simulink model "PII_speed"  (Simulink 7.5)
settings: Solver=ode1  SolverMode=SingleTasking  StartTime=0.0  StopTime=Inf  FixedStep=ts  RelTol=1e-3
PostLoadFcn:
  | , if any(exist('dsrtsu_mdlpostloadfcn', 'file') == [2, 3, 6]), try dsrtsu_mdlpostloadfcn('Execute', bdroot); catch fprintf('Error in PostLoadFcn (dsrtsu_mdlpostloadfcn) for model "%s":\n %s\n', bdroot, lasterr); end, end,
values from neighbouring files (symbols this model uses):
  Amp = 0    [RUN.m]
  en = 0    [RUN.m]
  f = 0.20    (= 0.2)    [RUN.m]
  g = 1    [RUN.m]
  kii = 660    [RUN.m]
  kpi = 2.0    (= 2)    [RUN.m]
  limit = 1    [RUN.m]
  nap = 0    [RUN.m]
  obc_del = 0.7    [RUN.m]
  obc_del2 = 1.3    [RUN.m]
  obc_en = 0    [RUN.m]
  obc_en1 = 0    [RUN.m]
  offset = 0    [RUN.m]
  res = 1    [RUN.m]
  res1 = 1    [RUN.m]
  start = 0    [RUN.m]
  Tf = 0.01    [RUN.m]
  Ts_i = 0.0002    [RUN.m]
  Ts_w = 0.001    [RUN.m]
undefined symbols (not defined in the file or in its folder): k1_singletons, k1k, k2_singletons, k2k, k3_singletons, k3k, kdu, Ki_singletons, Kik, ku, mf
libraries: fuzblock x15, rtilib1103 x6, simulink_extras x1
(part 1 of 2)
settings Model: DSRTSU_INTERNAL_RTI_VER=400  DSRTSU_INTERNAL_RTI_TYPE=rti1103  Creator=lab108  LastModifiedBy=zychlewicz  TunableVars=Amp,Q,Start,en,f,g,kii,kpi,n_max,n_min,nap,nb_nb,obc_del,obc_del2,obc_en,obc_en1,obc_poz,offset,p_gain,skal_u,start  TunableVarsStorageClass=Auto,Auto,Auto,Auto,Auto,Auto,Auto,Auto,Auto,Auto,Auto,Auto,Auto,Auto,Auto,Auto,Auto,Auto,Auto,Auto,Auto  TunableVarsTypeQualifier=,,,,,,,,,,,,,,,,,,,,  BufferReuse=off
settings OptimizationCC: BlockReduction=off  InlineParams=on  OptimizeBlockIOStorage=off  BufferReuse=off  ExpressionFolding=off  LocalBlockOutputs=off
settings DebuggingCC: StrictBusMsg=Warning
settings HardwareCC: ProdIntDivRoundTo=Zero  ProdEndianess=BigEndian  ProdHWDeviceType=Generic->Custom  TargetIntDivRoundTo=Zero  TargetEndianess=BigEndian  TargetHWDeviceType=Generic->Custom
settings RTWCC: SystemTargetFile=rti1103.tlc  MakeCommand=make_rti  TemplateMakefile=rti1103.tmf  Description=dSPACE DS1103 Hardware Platform  ProcessScript=rti1103_make_rtw_hook
settings STFCustomTargetCC: ParMdlRefBuildCompliant=on  GeneratePreprocessorConditionals=Disable all  SystemTargetFile=rti1103.tlc
settings GRTTargetCC: CompOptLevelCompliant=off  MatFileLogging=off  ExtModeMexFile=noextcomm
settings CustomProperty: DataType=RTWOptions_EnumType_D__dSPACE RCPHIL 73_matlab_rti1103_tlc_rti1103_1InitialSimState  Value=RUN
settings EnumStrPairs: String=RUN
settings SimEventsCC: propDiagAttribOutput=1  propDiagFcnCallOutput=1  propDiagStatOutput=0

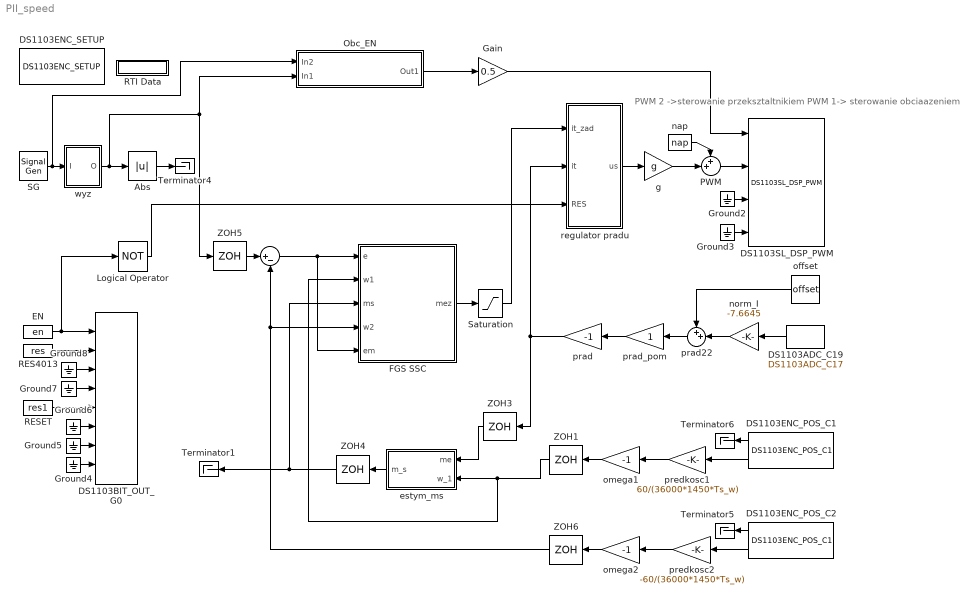
== system PII_speed ==
  note: PWM 2 ->sterowanie przeksztaltnikiem
      | PWM 1-> sterowanie obciaazeniem
  " " : Sum  Inputs=|+-  OutDataType=sfix(16)  OutScaling=2^0
  Abs : Abs  OutDataType=fixdt(1, 16)  OutScaling=2^0
  DS1103ADC_C19 : rtilib1103/DS1103 MASTER PPC/DS1103ADC_C17  SystemSampleTime=-1  ChannelNo=19  TimerAPreTrigger=0  Reserved2=[]  Reserved3=[]  Reserved4=[]  DialogFcn=gui1103adc  UnitName={ 'DS1103ADC_C' }  UnitValues={ 19 }  DSProperties=struct('RTI',struct('Version',uint32(1),'BlockType',struct('isSLSource',uint8(1),'isSLSink',uint8(0),'isHWSource',uint8(1),'isHWSink',uint8(0),'isSetup',uint8(0),'isInline',uint8(1),'isNonInline',uint8(0),'isInterrupt',uint8(0),'isChannelwise',uint8(1)),'IOBoardType','DS1103MASTER','UnitType','ADC','Identifier','ADC','DialogType','ML','BlockSet','NONE','SlaveProcessor','NONE'))
  DS1103BIT_OUT_G0 : rtilib1103/DS1103 MASTER PPC/DS1103BIT_OUT_G0  SystemSampleTime=-1  GroupNo=0  InitValue=[0 0 0 0 0 0 0 0]  TermMode=[1 1 1 1 1 1 1 1]  TermValue=[0 0 0 0 0 0 0 0]  Reserved1=[]  Reserved2=[]  Reserved3=[]  Reserved=[]  DialogFcn=gui1103bit_out  UnitName={ 'DS1103BIT_OUT_G'}  UnitValues={ 0 }  DSProperties=struct('RTI',struct('Version',uint32(1),'BlockType',struct('isSLSource',uint8(0),'isSLSink',uint8(1),'isHWSource',uint8(0),'isHWSink',uint8(1),'isSetup',uint8(0),'isInline',uint8(1),'isNonInline',uint8(0),'isInterrupt',uint8(0),'isChannelwise',uint8(0)),'IOBoardType','DS1103MASTER','UnitType','BIT','Identifier','BITOUT','DialogType','ML','BlockSet','NONE','SlaveProcessor','NONE'))
  DS1103ENC_POS_C1 : rtilib1103/DS1103 MASTER PPC/DS1103ENC_POS_C1  SystemSampleTime=-1  ChannelNo=1  PosValue=0  Reserved1=[]  Reserved2=[]  Reserved3=[]  Reserved4=[]  DialogFcn=gui1103enc_pos  UnitName={ 'DS1103ENC_POS_C' }  UnitValues={ 1 }  DSProperties=struct('RTI',struct('Version',uint32(1),'BlockType',struct('isSLSource',uint8(1),'isSLSink',uint8(0),'isHWSource',uint8(1),'isHWSink',uint8(0),'isSetup',uint8(0),'isInline',uint8(1),'isNonInline',uint8(0),'isInterrupt',uint8(0),'isChannelwise',uint8(1)),'IOBoardType','DS1103MASTER','UnitType','ENC','Identifier','ENCPOSCH','DialogType','ML','BlockSet','NONE','SlaveProcessor','NONE'))
  DS1103ENC_POS_C2 : rtilib1103/DS1103 MASTER PPC/DS1103ENC_POS_C1  SystemSampleTime=-1  ChannelNo=2  PosValue=0  Reserved1=[]  Reserved2=[]  Reserved3=[]  Reserved4=[]  DialogFcn=gui1103enc_pos  UnitName={ 'DS1103ENC_POS_C' }  UnitValues={2}  DSProperties=struct('RTI',struct('Version',uint32(1),'BlockType',struct('isSLSource',uint8(1),'isSLSink',uint8(0),'isHWSource',uint8(1),'isHWSink',uint8(0),'isSetup',uint8(0),'isInline',uint8(1),'isNonInline',uint8(0),'isInterrupt',uint8(0),'isChannelwise',uint8(1)),'IOBoardType','DS1103MASTER','UnitType','ENC','Identifier','ENCPOSCH','DialogType','ML','BlockSet','NONE','SlaveProcessor','NONE'))
  DS1103ENC_SETUP : rtilib1103/DS1103 MASTER PPC/DS1103ENC_SETUP  SystemSampleTime=-1  EncRange=2  Reserved1=[]  Reserved2=[]  Reserved3=[]  Reserved4=[]  DialogFcn=gui1103enc_setup  UnitName={ 'DS1103ENC_SETUP' }  UnitValues={ [] }  DSProperties=struct('RTI',struct('Version',uint32(1),'BlockType',struct('isSLSource',uint8(0),'isSLSink',uint8(0),'isHWSource',uint8(0),'isHWSink',uint8(0),'isSetup',uint8(0),'isInline',uint8(1),'isNonInline',uint8(0),'isInterrupt',uint8(0),'isChannelwise',uint8(0)),'IOBoardType','DS1103MASTER','UnitType','ENC','Identifier','ENCMASTER','DialogType','ML','BlockSet','NONE','SlaveProcessor','NONE'))
      settings: SignalType=[1 1 1 1 1 1 0]
  DS1103SL_DSP_PWM : rtilib1103/DS1103 SLAVE DSP/DS1103SL_DSP_PWM  SystemSampleTime=-1  Parameters=[]  TDef=[]  BoardType=[]  PwmMode=[]  Frequency=[]  InitValue=[]  TermMode=[]  TermValue=[]  Polarity=[]  DialogFcn=[]  Reserved1=[]  Reserved2=[]  Reserved3=[]  Reserved4=[]  Revision=[]  UnitName=[]  UnitValues=[]  DSProperties=struct('RTI',struct('Version',uint32(2),'BlockType',struct('isSLSource',uint8(0),'isSLSink',uint8(1),'isHWSource',uint8(0),'isHWSink',uint8(1),'isSetup',uint8(0),'isInline',uint8(1),'isNonInline',uint8(0),'isInterrupt',uint8(0),'isChannelwise',uint8(0)),'IOBoardType','DS1103SLAVE','UnitType','PWM','Identifier','PWM','DialogType','ML','BlockSet','NONE','SlaveProcessor','F240'))  RTIBlockInterface=struct('InputPortsActive',[1 1 1 1],'InputPortsWidth',int32([2 1 2 2]),'InputPortsName',{{['PWM Channel 1'],['PWM Channel 2'],['PWM Channel 3'],['PWM Channel 4']}},'IWork',{{{'',uint32(4)}}},'DialogFcn','rti1103slavepwmgui','InitLevel',1,'BlockDisplay',{{'','auto'}},'IconTransparency','on','MultiSFcn',4,'BlockName',struct('Token',{{'DS1103SL_DSP_PWM'}}))  RTIBlockParameters=struct('PWMSymmetryMode',{{1,'OFF',[]}},'PWMFrequency',{{'12000','OFF',[]}},'PWMPolarityMode',{{[1 1 1 1 1],'OFF',[]}},'ChannelNo',{{[1 2 3 4],'OFF',[]}},'SuspendModeInit',{{[1 0 1 1 1],'OFF',[]}},'TTLModeInit',{{[2 2 2 2 2],'OFF',[]}},'DutyCycleInitValueCh1',{{'0.5','OFF',[]}},'DutyCycleInitValueCh2',{{'0.5','OFF',[]}},'DutyCycleInitValueCh3',{{'0.5','OFF',[]}},'DutyCycleInitValueCh4',{{'0.5','OFF',[]}},'DutyCycleInitValueCh5',{{'0.5','OFF',[]}},'EnablePWMStop',{{[1 1 1 1 0],'OFF',[]}},'SuspendModeTerm',{{[1 0 1 1 1],'OFF',[]}},'TTLModeTerm',{{[2 2 2 2 2],'OFF',[]}},'DutyCycleTermValueCh1',{{'0.5','OFF',[]}},'DutyCycleTermValueCh2',{{'0.5','OFF',[]}},'DutyCycleTermValueCh3',{{'0.5','OFF',[]}},'DutyCycleTermValueCh4',{{'0.5','OFF',[]}},'DutyCycleTermValueCh5',{{'0.5','OFF',[]}},'TLCFileName',{{'rti1103pwm','OFF',[]}})  RTISFcnParameters=struct('PWMSymmetryMode','double','PWMFrequency','double','PWMPolarityMode','double','ChannelNo','double','SuspendModeInit','double','TTLModeInit','double','DutyCycleInitValueCh1','double','DutyCycleInitValueCh2','double','DutyCycleInitValueCh3','double','DutyCycleInitValueCh4','double','EnablePWMStop','double','SuspendModeTerm','double','TTLModeTerm','double','DutyCycleTermValueCh1','double','DutyCycleTermValueCh2','double','DutyCycleTermValueCh3','double','DutyCycleTermValueCh4','double','TLCFileName','char')  RTIBlockParaDefault=struct('PWMSymmetryMode',1,'PWMFrequency',100,'PWMPolarityMode',[1 1 1 1 1],'ChannelNo',[1 2 3 4],'SuspendModeInit',[1 1 1 1 1],'TTLModeInit',[2 2 2 2 2],'DutyCycleInitValueCh1',0.5,'DutyCycleInitValueCh2',0.5,'DutyCycleInitValueCh3',0.5,'DutyCycleInitValueCh4',0.5,'DutyCycleInitValueCh5',0.5,'EnablePWMStop',[1 1 1 1 0],'SuspendModeTerm',[1 1 1 1 1],'TTLModeTerm',[2 2 2 2 2],'DutyCycleTermValueCh1',0.5,'DutyCycleTermValueCh2',0.5,'DutyCycleTermValueCh3',0.5,'DutyCycleTermValueCh4',0.5,'DutyCycleTermValueCh5',0.5,'TLCFileName','rti1103pwm')
  EN : Constant  Value=en  OutDataTypeMode=boolean  OutDataType=fixdt(1, 16)  OutScaling=2^0  OutDataTypeStr=boolean
  FGS SSC : Subsystem
      mask Display:
      | port_label('input', 1, 'error', 'texmode', 'on')
      | port_label('input', 2, '\omega_1', 'texmode', 'on')
      | port_label('input', 3, 'm_s', 'texmode', 'on')
      | port_label('input', 4, '\omega_2', 'texmode', 'on')
      | port_label('input', 5, '\omega_{refm} - \omega_1', 'texmode', 'on')
      | port_label('output', 1, 'm_{ez}', 'texmode', 'on')
      | color('red')
      | disp('FGS SSC')
      | color('blue')
      | plot(gaussmf([-1:0.0001:1],[1 0]))
  Gain : Gain  Gain=0.5  ParameterDataType=sfix(16)  ParameterScaling=2^0  OutDataType=sfix(16)  OutScaling=2^0
  Ground{2..8} (7 alike) : Ground
  Logical Operator : Logic  Operator=NOT  AllPortsSameDT=off  OutDataTypeMode=boolean  LogicDataType=fixdt(0, 8)  OutDataTypeStr=boolean
  Obc_EN : Subsystem
  PWM : Sum  Inputs=++|  OutDataType=sfix(16)  OutScaling=2^0
  RES4013 : Constant  Value=res  OutDataTypeMode=boolean  OutDataType=fixdt(1, 16)  OutScaling=2^0  OutDataTypeStr=boolean
  RESET : Constant  Value=res1  OutDataTypeMode=boolean  OutDataType=fixdt(1, 16)  OutScaling=2^0  OutDataTypeStr=boolean
  RTI Data : Subsystem  Tag=struct('RTIDataServer',struct('RTIDataServerVs','2','RTIModelDescription','struct(''main'',''PII_speed'',''sub'','''',''isMp'',0)'))  LoadFcn="if exist('rtidc'), try,  rtidc('DataHostBlockClbLoad', gcbh); catch, disp(['Warning: ''LoadFcn'' for RTI Data block failed: ' lasterr]); end, end,"
      settings: CopyFcn="if exist('rtidc'), try,  rtidc('DataHostBlockClbCopy', gcbh); catch, disp(['Warning: ''CopyFcn'' for RTI Data block failed: ' lasterr]); end, end,"  DeleteFcn="if exist('rtidc'), try,  rtidc('DataHostBlockClbDelete', gcbh); catch, disp(['Warning: ''DeleteFcn'' for RTI Data block failed: ' lasterr]); end, end,"  ModelCloseFcn="if exist('rtidc'), try,  rtidc('DataHostBlockClbModelClose', gcbh); catch, disp(['Warning: ''ModelCloseFcn'' for RTI Data block failed: ' lasterr]); end, end,"  PreSaveFcn="if exist('rtidc'), try,  rtidc('DataHostBlockClbPreSave', gcbh); catch, disp(['Warning: ''PreSaveFcn'' for RTI Data block failed: ' lasterr]); end, end,"  PostSaveFcn="if exist('rtidc'), try,  rtidc('DataHostBlockClbPostSave', gcbh); catch, disp(['Warning: ''PostSaveFcn'' for RTI Data block failed: ' lasterr]); end, end,"  NameChangeFcn="if exist('rtidc'), try,  rtidc('DataHostBlockClbNameChange', gcbh); catch, disp(['Warning: ''NameChangeFcn'' for RTI Data block failed: ' lasterr]); end, end,"
      mask Type: RTI_DATA_HOST
      mask Description:
      | RTI Data Block.
      | This block is used by RTI to store internal model-dependent data.
      | Please keep this block on the root level of the model. Deleting this block will result in data loss.
      | 
      | NEVER DELETE OR COPY THIS BLOCK!
      mask Help:
      | RTI Data Block.
      | This block is used by RTI to store internal model-dependent data.
      | Please keep this block on the root level of the model. Deleting this block will result in data loss.
      | 
      | NEVER DELETE OR COPY THIS BLOCK!
      mask Display:
      | text(0.5, 0.5, 'RTI Data', 'HorizontalAlignment', 'center');
      | plot([1 0]);
  SG : SignalGenerator  WaveForm=square  Amplitude=Amp  Frequency=f
  Saturation : Saturate  UpperLimit=limit  LowerLimit=-limit
  Terminator{1,4..6} (4 alike) : Terminator
  ZOH{1,3..6} (5 alike) : ZeroOrderHold  SampleTime=Ts_w
  estym_ms : Subsystem
  g : Gain  Gain=g  ParameterDataType=fixdt(1, 16)  ParameterScaling=2^0  OutDataType=fixdt(1, 16)  OutScaling=2^0
  nap : Constant  Value=nap  OutDataType=sfix(16)  OutScaling=2^0
  norm_I : Gain  Gain=-7.6645  ParameterDataType=fixdt(1, 16)  ParameterScaling=2^0  OutDataType=fixdt(1, 16)  OutScaling=2^0
  offset : Constant  Value=offset  OutDataType=sfix(16)  OutScaling=2^0
  omega1 : Gain  Gain=-1  OutDataTypeMode=double  OutDataTypeStr=double  SampleTime=Ts_w  SaturateOnIntegerOverflow=on  ParamDataTypeStr=Inherit: Same as input
  omega2 : Gain  Gain=-1  OutDataTypeMode=double  OutDataTypeStr=double  SampleTime=Ts_w  SaturateOnIntegerOverflow=on  ParamDataTypeStr=Inherit: Same as input
  prad : Gain  Gain=-1  OutDataTypeMode=double  OutDataTypeStr=double  SampleTime=Ts_i  SaturateOnIntegerOverflow=on  ParamDataTypeStr=Inherit: Same as input
  prad22 : Sum  Inputs=++|  OutDataType=sfix(16)  OutScaling=2^0
  prad_pom : Gain  OutDataTypeMode=double  OutDataTypeStr=double  SampleTime=Ts_i  SaturateOnIntegerOverflow=on  ParamDataTypeStr=Inherit: Same as input
  predkosc1 : Gain  Gain=60/(36000*1450*Ts_w)  OutDataTypeMode=double  OutDataTypeStr=double  SampleTime=Ts_w  SaturateOnIntegerOverflow=on  ParamDataTypeStr=Inherit: Same as input
  predkosc2 : Gain  Gain=-60/(36000*1450*Ts_w)  OutDataTypeMode=double  OutDataTypeStr=double  SampleTime=Ts_w  SaturateOnIntegerOverflow=on  ParamDataTypeStr=Inherit: Same as input
  regulator pradu : Subsystem
  wyz : Subsystem
  wires:
  EN/1 -> DS1103BIT_OUT_G0/1, Logical Operator/1
  RESET/1 -> DS1103BIT_OUT_G0/5
  RES4013/1 -> DS1103BIT_OUT_G0/2
  DS1103ADC_C19/1 -> norm_I/1
  offset/1 -> prad22/1
  norm_I/1 -> prad22/2
  DS1103ENC_POS_C1/2 -> predkosc1/1
  prad22/1 -> prad_pom/1
  DS1103ENC_POS_C2/2 -> predkosc2/1
  nap/1 -> PWM/1
  regulator pradu/1(us) -> g/1
  PWM/1 -> DS1103SL_DSP_PWM/2
  g/1 -> PWM/2
  SG/1 -> wyz/1(I), Obc_EN/1(In2)
  predkosc2/1 -> omega2/1
  predkosc1/1 -> omega1/1
  wyz/1(O) -> Abs/1, Obc_EN/2(In1), ZOH5/1
  Ground2/1 -> DS1103SL_DSP_PWM/3
  Ground3/1 -> DS1103SL_DSP_PWM/4
  Ground4/1 -> DS1103BIT_OUT_G0/8
  Ground5/1 -> DS1103BIT_OUT_G0/7
  Ground6/1 -> DS1103BIT_OUT_G0/6
  Ground7/1 -> DS1103BIT_OUT_G0/4
  Ground8/1 -> DS1103BIT_OUT_G0/3
  Abs/1 -> Terminator4/1
  DS1103ENC_POS_C2/1 -> Terminator5/1
  DS1103ENC_POS_C1/1 -> Terminator6/1
  Logical Operator/1 -> regulator pradu/3(RES)
  prad/1 -> regulator pradu/2(it), ZOH3/1
  Obc_EN/1(Out1) -> Gain/1
  Gain/1 -> DS1103SL_DSP_PWM/1
  ZOH3/1 -> estym_ms/1(me)
  omega1/1 -> ZOH1/1
  ZOH1/1 -> estym_ms/2(w_1), FGS SSC/2(w1)
  prad_pom/1 -> prad/1
  omega2/1 -> ZOH6/1
  estym_ms/1(m_s) -> ZOH4/1
  Saturation/1 -> regulator pradu/1(it_zad)
  FGS SSC/1(mez) -> Saturation/1
  ZOH4/1 -> Terminator1/1, FGS SSC/3(ms)
  ZOH6/1 -> FGS SSC/4(w2), " "/2
  ZOH5/1 -> " "/1
  " "/1 -> FGS SSC/1(e), FGS SSC/5(em)

== system PII_speed/FGS SSC ==
  e : Inport
  w1 : Inport  Port=2
  ms : Inport  Port=3
  w2 : Inport  Port=4
  em : Inport  Port=5
  FGS : Subsystem
      mask Display:
      | port_label('output',1,'K_i^{fuzzy}','texmode','on')
      | port_label('output',2,'k_1^{fuzzy}','texmode','on')
      | port_label('output',3,'k_2^{fuzzy}','texmode','on')
      | port_label('output',4,'k_3^{fuzzy}','texmode','on')
      | port_label('input',1,'error','texmode','on')
  Integrator : Integrator
  Product{1..2,5..6} (4 alike) : Product
  Sum1 : Sum  Inputs=++|
  Sum7 : Sum  Inputs=|+-
  Sum9 : Sum  Inputs=++|
  mez : Outport
  wires:
  Sum9/1 -> Sum7/2
  Sum1/1 -> Sum9/2
  Product6/1 -> Sum1/2
  Product2/1 -> Sum9/1
  w2/1 -> Product6/1
  ms/1 -> Product5/1
  w1/1 -> Product2/1
  Sum7/1 -> mez/1
  Product1/1 -> Sum7/1
  Integrator/1 -> Product1/1
  e/1 -> Integrator/1
  Product5/1 -> Sum1/1
  em/1 -> FGS/1(e)
  FGS/1(Kifuzzy) -> Product1/2
  FGS/2(k1fuzzy) -> Product2/2
  FGS/4(k3fuzzy) -> Product6/2
  FGS/3(k2fuzzy) -> Product5/2

== system PII_speed/Obc_EN ==
  In2 : Inport
  In1 : Inport  Port=2
  Abs : Abs  OutDataType=fixdt(1, 16)  OutScaling=2^0
  Add : Sum  Inputs=+-  OutDataType=fixdt(1, 16)  OutScaling=2^-10
  Bus Creator : BusCreator  Inputs=2
  Gain : Gain  Gain=-1  ParameterDataType=sfix(16)  ParameterScaling=2^0  OutDataType=sfix(16)  OutScaling=2^0
  Obc_en : Step  Time=0  After=obc_en  SampleTime=0
  Obc_en1 : Step  Time=0  After=obc_en1  SampleTime=0
  Obc_poziom : Lookup  InputValues=[0,0.25,0.3,0.4,0.5,0.6,0.75,1]  Table=[-1,-1,-0.78,-0.4,-0.3,-0.24,-0.18,-0.13]  OutDataType=fixdt(1, 16)  OutScaling=2^0
  Product : Product  Inputs=3  OutDataType=sfix(16)  OutScaling=2^0  RndMeth=Zero
  Sign : Signum
  Sign1 : Signum
  TD : TransportDelay  DelayTime=obc_del  BufferSize=60000
  TD1 : TransportDelay  DelayTime=obc_del2  BufferSize=60000
  Out1 : Outport
  wires:
  Obc_en/1 -> Product/1
  Product/1 -> Bus Creator/1
  In1/1 -> Gain/1
  Bus Creator/1 -> Out1/1
  TD/1 -> Sign/1, TD1/1
  Sign/1 -> Add/1
  Gain/1 -> TD/1
  TD1/1 -> Sign1/1
  Sign1/1 -> Add/2
  Add/1 -> Product/2
  Abs/1 -> Obc_poziom/1
  Obc_poziom/1 -> Product/3
  In2/1 -> Abs/1
  Obc_en1/1 -> Bus Creator/2

== system PII_speed/RTI Data ==
  RTI Data Store : Subsystem  Tag="struct('private',struct('version',struct('dsVer',uint32(2),'dsVerCreation',uint32(2),'RTI',struct('ver','6.4','type','RTI1103')),'access',struct('type','Model','isPerm',1,'created',['17-Sep-2010 12:08:45'],'modified',['21-Jan-2016 14:22:11'],'location','')),'public',struct('main',struct('data',[]),'sub',struct('name',{{'PII_speed'}},'data',{{struct('TH',struct('thTaskInfo',struct('taskType',{'TIMER','HWINT','TMRINT','SWINT','GLINT'},'tasksNumOf',{1,0,0,0,0},'srcIds',{{'TIMERA'},{},{},{},{}},'taskNames',{{['Timer Task 1']},{},{},{},{}})),'th_tc',struct('dataType','TASK','taskGroupId','','taskGroupList',{{}},'taskSchedulingPolicy','FCFS','taskType','TIMER','blkh',-1,'srcId','TIMERA','srcSgnName',['Timer A interrupt'],'srcCpuName','','taskName',['Timer Task 1  [0.0001] s'],'taskNameDisplayExt','','smplTime',0.0001,'smplTimeOffs',0,'hasFixedPriority',0,'priority',1,'hasFixedOvc',0,'ovcType',1,'ovcMax',1),'tc_th',struct('dataType','TASK','taskGroupId','','taskGroupList',{{}},'taskSchedulingPolicy','FCFS','taskType','TIMER','blkh',-1,'srcId','TIMERA','srcSgnName',['Timer A interrupt'],'srcCpuName','','taskName',['Timer Task 1  [0.0001] s'],'taskNameDisplayExt','','smplTime',0.0001,'smplTimeOffs',0,'hasFixedPriority',0,'priority',1,'hasFixedOvc',0,'ovcType',1,'ovcMax',1))}})))"
      mask Type: RTI_DATA_STORE
      mask Description:
      | RTI Data Store Block. This block is used by RTI to store internal model dependent data. Deleting this block will result in data loss.
      | 
      | NEVER DELETE, COPY, OR MODIFY THIS BLOCK!
      mask Help:
      | RTI Data Store Block. This block is used by RTI to store internal model dependent data. Deleting this block will result in data loss.
      | 
      | NEVER DELETE, COPY, OR MODIFY THIS BLOCK!
      mask Display: text(0.5, 0.5, ' ', 'HorizontalAlignment', 'center');

== system PII_speed/estym_ms ==
  me : Inport
  w_1 : Inport  Port=2
  Transfer Fcn1 : TransferFcn  Numerator=[0.203 0]  Denominator=[Tf 1]
  Transfer Fcn2 : TransferFcn  Denominator=[Tf 1]
  ms_est : Sum  Inputs=-+  OutDataType=sfix(16)  OutScaling=2^0
  m_s : Outport
  wires:
  ms_est/1 -> m_s/1
  me/1 -> Transfer Fcn2/1
  w_1/1 -> Transfer Fcn1/1
  Transfer Fcn2/1 -> ms_est/2
  Transfer Fcn1/1 -> ms_est/1

== system PII_speed/regulator pradu ==
  it_zad : Inport  SampleTime=Ts_i
  it : Inport  Port=2  SampleTime=Ts_i
  RES : Inport  Port=3  SampleTime=Ts_i
  Continous-time integrator : Integrator  ExternalReset=level  LimitOutput=on  UpperSaturationLimit=0.52  LowerSaturationLimit=-0.52
  KI : Gain  Gain=kii  SampleTime=Ts_i  SaturateOnIntegerOverflow=on  OutDataTypeStr=Inherit: Same as input  ParamDataTypeStr=Inherit: Same as input
  Kp : Gain  Gain=kpi  SampleTime=Ts_i  SaturateOnIntegerOverflow=on  OutDataTypeStr=Inherit: Same as input  ParamDataTypeStr=Inherit: Same as input
  Saturation : Saturate  UpperLimit=0.52  LowerLimit=-0.52  OutDataType=fixdt(1, 16)  OutScaling=2^0
  Sum1 : Sum  Inputs=|+-  SampleTime=Ts_i  SaturateOnIntegerOverflow=on  InputSameDT=on  OutDataTypeStr=Inherit: Same as first input
  Sum2 : Sum  SampleTime=Ts_i  SaturateOnIntegerOverflow=on  InputSameDT=on  OutDataTypeStr=Inherit: Same as first input
  offset : Constant  Value=0.5  OutDataType=sfix(16)  OutScaling=2^0  SampleTime=Ts_i
  prad : Sum  Inputs=++|  OutDataType=sfix(16)  OutScaling=2^0  SampleTime=Ts_i
  us : Outport
  wires:
  Kp/1 -> Sum2/1
  Sum2/1 -> Saturation/1
  Sum1/1 -> Kp/1, KI/1
  it/1 -> Sum1/2
  it_zad/1 -> Sum1/1
  RES/1 -> Continous-time integrator/2
  offset/1 -> prad/1
  prad/1 -> us/1
  KI/1 -> Continous-time integrator/1
  Continous-time integrator/1 -> Sum2/2
  Saturation/1 -> prad/2

== system PII_speed/wyz ==
  I : Inport
  HC : HitCross  HitCrossingDirection=rising
  LO : Logic  AllPortsSameDT=off  OutDataTypeMode=boolean  LogicDataType=fixdt(0, 8)  OutDataTypeStr=boolean
  LO3 : Logic  Operator=NOT  AllPortsSameDT=off
  S : Constant  Value=0  OutDataTypeMode=boolean  OutDataTypeStr=boolean
  S-R Flip-Flop : simulink_extras/Flip Flops/S-R Flip-Flop  SystemSampleTime=-1  initial_condition=0
  Start : Constant  Value=start
  Switch : Switch  Criteria=u2 ~= 0  OutDataType=fixdt(1, 16)  OutScaling=2^0
  Terminator5 : Terminator
  O : Outport
  wires:
  Start/1 -> LO3/1, LO/2
  HC/1 -> LO/1
  LO/1 -> S-R Flip-Flop/1
  LO3/1 -> S-R Flip-Flop/2
  Switch/1 -> O/1
  S/1 -> Switch/3
  S-R Flip-Flop/1 -> Switch/2
  I/1 -> HC/1, Switch/1
  S-R Flip-Flop/2 -> Terminator5/1

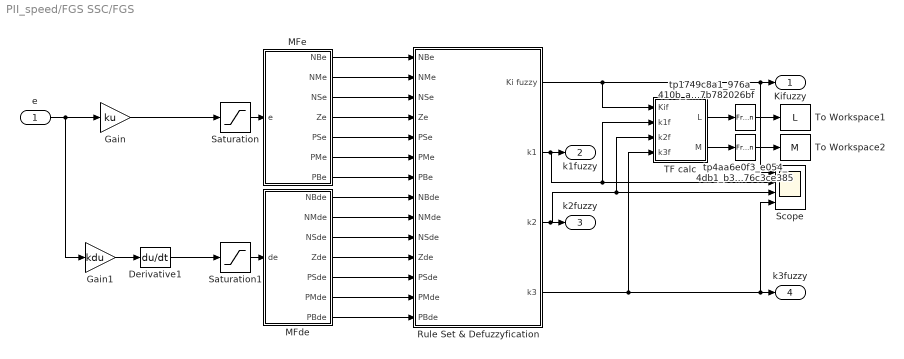
== system PII_speed/FGS SSC/FGS ==
  e : Inport
  Derivative1 : Derivative
  Gain : Gain  Gain=ku
  Gain1 : Gain  Gain=kdu
  MFde : Subsystem
  MFe : Subsystem
  Rule Set & Defuzzyfication : Subsystem
  Saturation : Saturate  UpperLimit=1  LowerLimit=-1
  Saturation1 : Saturate  UpperLimit=1  LowerLimit=-1
  Scope : Scope  NumInputPorts=4
      settings: TimeRange=20  YMin=27.01~10.375~2.85~0.061  YMax=27.08~10.42~3.2~0.0655  SaveName=data2  DataFormat=Array
  TF calc : Subsystem
  To Workspace1 : ToWorkspace  VariableName=L  SampleTime=-1  SaveFormat=Array
  To Workspace2 : ToWorkspace  VariableName=M  SampleTime=-1  SaveFormat=Array
  tp1749c8a1_976a_410b_a3f7_9c7b782026bf : FrameConversion  OutFrame=Sample-based
  tp4aa6e0f3_e054_4db1_b332_b1b76c3ce385 : FrameConversion
  Kifuzzy : Outport
  k1fuzzy : Outport  Port=2
  k2fuzzy : Outport  Port=3
  k3fuzzy : Outport  Port=4
  wires:
  Rule Set & Defuzzyfication/1(Ki fuzzy) -> TF calc/1(Kif), Kifuzzy/1, Scope/1
  MFde/7(PBde) -> Rule Set & Defuzzyfication/14(PBde)
  MFde/6(PMde) -> Rule Set & Defuzzyfication/13(PMde)
  MFde/5(PSde) -> Rule Set & Defuzzyfication/12(PSde)
  MFde/4(Zde) -> Rule Set & Defuzzyfication/11(Zde)
  MFde/3(NSde) -> Rule Set & Defuzzyfication/10(NSde)
  MFde/2(NMde) -> Rule Set & Defuzzyfication/9(NMde)
  MFde/1(NBde) -> Rule Set & Defuzzyfication/8(NBde)
  MFe/7(PBe) -> Rule Set & Defuzzyfication/7(PBe)
  MFe/6(PMe) -> Rule Set & Defuzzyfication/6(PMe)
  MFe/5(PSe) -> Rule Set & Defuzzyfication/5(PSe)
  MFe/4(Ze) -> Rule Set & Defuzzyfication/4(Ze)
  MFe/3(NSe) -> Rule Set & Defuzzyfication/3(NSe)
  MFe/2(NMe) -> Rule Set & Defuzzyfication/2(NMe)
  MFe/1(NBe) -> Rule Set & Defuzzyfication/1(NBe)
  Gain/1 -> Saturation/1
  e/1 -> Gain/1, Gain1/1
  Rule Set & Defuzzyfication/3(k2) -> Scope/3, TF calc/3(k2f), k2fuzzy/1
  Rule Set & Defuzzyfication/4(k3) -> Scope/4, k3fuzzy/1, TF calc/4(k3f)
  Rule Set & Defuzzyfication/2(k1) -> Scope/2, TF calc/2(k1f), k1fuzzy/1
  Saturation/1 -> MFe/1(e)
  Saturation1/1 -> MFde/1(de)
  Gain1/1 -> Derivative1/1
  Derivative1/1 -> Saturation1/1
  TF calc/1(L) -> tp1749c8a1_976a_410b_a3f7_9c7b782026bf/1
  tp1749c8a1_976a_410b_a3f7_9c7b782026bf/1 -> To Workspace1/1
  TF calc/2(M) -> tp4aa6e0f3_e054_4db1_b332_b1b76c3ce385/1
  tp4aa6e0f3_e054_4db1_b332_b1b76c3ce385/1 -> To Workspace2/1

== system PII_speed/RTI Data/RTI Data Store ==
  RTI Data Store : Subsystem
      mask Type: RTI_DATA_STORE
      mask Description:
      | RTI Data Store Block. This block is used by RTI to store internal model dependent data. Deleting this block will result in data loss.
      | 
      | NEVER DELETE, COPY, OR MODIFY THIS BLOCK!
      mask Help:
      | RTI Data Store Block. This block is used by RTI to store internal model dependent data. Deleting this block will result in data loss.
      | 
      | NEVER DELETE, COPY, OR MODIFY THIS BLOCK!
      mask Display: text(0.5, 0.5, ' ', 'HorizontalAlignment', 'center');

== system PII_speed/FGS SSC/FGS/MFde ==
  de : Inport
  Gaussian MF : fuzblock/Membership  Functions/Gaussian MF  sigma=sigma  mu=mf(1)
  Gaussian MF1 : fuzblock/Membership  Functions/Gaussian MF  sigma=sigma  mu=mf(2)
  Gaussian MF2 : fuzblock/Membership  Functions/Gaussian MF  sigma=sigma  mu=mf(3)
  Gaussian MF3 : fuzblock/Membership  Functions/Gaussian MF  sigma=sigma  mu=mf(4)
  Gaussian MF4 : fuzblock/Membership  Functions/Gaussian MF  sigma=sigma  mu=mf(5)
  Gaussian MF5 : fuzblock/Membership  Functions/Gaussian MF  sigma=sigma  mu=mf(6)
  Gaussian MF6 : fuzblock/Membership  Functions/Gaussian MF  sigma=sigma  mu=mf(7)
  NBde : Outport
  NMde : Outport  Port=2
  NSde : Outport  Port=3
  Zde : Outport  Port=4
  PSde : Outport  Port=5
  PMde : Outport  Port=6
  PBde : Outport  Port=7
  wires:
  Gaussian MF3/1 -> Zde/1
  de/1 -> Gaussian MF3/1, Gaussian MF2/1, Gaussian MF/1, Gaussian MF1/1, Gaussian MF4/1, Gaussian MF6/1, Gaussian MF5/1
  Gaussian MF2/1 -> NSde/1
  Gaussian MF5/1 -> PMde/1
  Gaussian MF4/1 -> PSde/1
  Gaussian MF6/1 -> PBde/1
  Gaussian MF1/1 -> NMde/1
  Gaussian MF/1 -> NBde/1

== system PII_speed/FGS SSC/FGS/MFe ==
  e : Inport
  Gaussian MF : fuzblock/Membership  Functions/Gaussian MF  SystemSampleTime=-1  sigma=sigma  mu=mf(1)
  Gaussian MF1 : fuzblock/Membership  Functions/Gaussian MF  SystemSampleTime=-1  sigma=sigma  mu=mf(2)
  Gaussian MF2 : fuzblock/Membership  Functions/Gaussian MF  SystemSampleTime=-1  sigma=sigma  mu=mf(3)
  Gaussian MF3 : fuzblock/Membership  Functions/Gaussian MF  SystemSampleTime=-1  sigma=sigma  mu=mf(4)
  Gaussian MF4 : fuzblock/Membership  Functions/Gaussian MF  SystemSampleTime=-1  sigma=sigma  mu=mf(5)
  Gaussian MF5 : fuzblock/Membership  Functions/Gaussian MF  SystemSampleTime=-1  sigma=sigma  mu=mf(6)
  Gaussian MF6 : fuzblock/Membership  Functions/Gaussian MF  SystemSampleTime=-1  sigma=sigma  mu=mf(7)
  Gaussian MF7 : fuzblock/Membership  Functions/Gaussian MF  SystemSampleTime=-1  sigma=1  mu=1
  NBe : Outport
  NMe : Outport  Port=2
  NSe : Outport  Port=3
  Ze : Outport  Port=4
  PSe : Outport  Port=5
  PMe : Outport  Port=6
  PBe : Outport  Port=7
  wires:
  Gaussian MF3/1 -> Ze/1
  e/1 -> Gaussian MF3/1, Gaussian MF2/1, Gaussian MF1/1, Gaussian MF/1, Gaussian MF4/1, Gaussian MF6/1, Gaussian MF5/1
  Gaussian MF2/1 -> NSe/1
  Gaussian MF5/1 -> PMe/1
  Gaussian MF4/1 -> PSe/1
  Gaussian MF6/1 -> PBe/1
  Gaussian MF1/1 -> NMe/1
  Gaussian MF/1 -> NBe/1

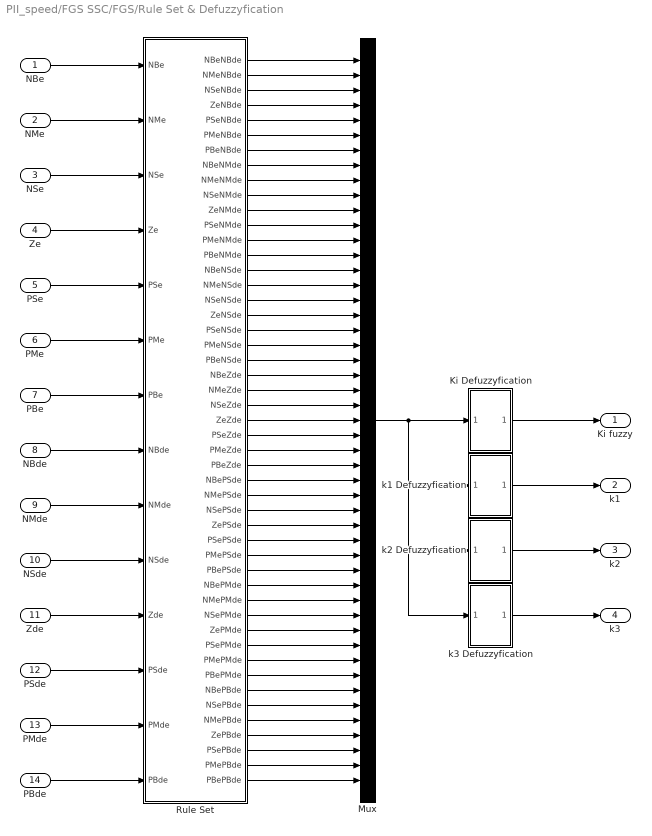
== system PII_speed/FGS SSC/FGS/Rule Set & Defuzzyfication ==
  NBe : Inport
  NMe : Inport  Port=2
  NSe : Inport  Port=3
  Ze : Inport  Port=4
  PSe : Inport  Port=5
  PMe : Inport  Port=6
  PBe : Inport  Port=7
  NBde : Inport  Port=8
  NMde : Inport  Port=9
  NSde : Inport  Port=10
  Zde : Inport  Port=11
  PSde : Inport  Port=12
  PMde : Inport  Port=13
  PBde : Inport  Port=14
  Ki Defuzzyfication : Subsystem
  Mux : Mux  Inputs=49
  Rule Set : Subsystem
  k1 Defuzzyfication : Subsystem
  k2 Defuzzyfication : Subsystem
  k3 Defuzzyfication : Subsystem
  Ki fuzzy : Outport
  k1 : Outport  Port=2
  k2 : Outport  Port=3
  k3 : Outport  Port=4
  wires:
  Mux/1 -> k1 Defuzzyfication/1(In1), k3 Defuzzyfication/1(In1), k2 Defuzzyfication/1(In1), Ki Defuzzyfication/1(In1)
  Rule Set/32(ZePSde) -> Mux/32
  Rule Set/43(NBePBde) -> Mux/43
  Rule Set/31(NSePSde) -> Mux/31
  Rule Set/33(PSePSde) -> Mux/33
  Rule Set/24(NSeZde) -> Mux/24
  Rule Set/46(ZePBde) -> Mux/46
  Rule Set/28(PBeZde) -> Mux/28
  Rule Set/49(PBePBde) -> Mux/49
  Rule Set/48(PMePBde) -> Mux/48
  Rule Set/39(ZePMde) -> Mux/39
  Rule Set/44(NSePBde) -> Mux/44
  Rule Set/35(PBePSde) -> Mux/35
  Rule Set/29(NBePSde) -> Mux/29
  Rule Set/40(PSePMde) -> Mux/40
  Rule Set/45(NMePBde) -> Mux/45
  Rule Set/27(PMeZde) -> Mux/27
  Rule Set/23(NMeZde) -> Mux/23
  Rule Set/25(ZeZde) -> Mux/25
  Rule Set/26(PSeZde) -> Mux/26
  Rule Set/34(PMePSde) -> Mux/34
  Rule Set/47(PSePBde) -> Mux/47
  Rule Set/37(NMePMde) -> Mux/37
  Rule Set/42(PBePMde) -> Mux/42
  Rule Set/41(PMePMde) -> Mux/41
  Rule Set/36(NBePMde) -> Mux/36
  Rule Set/30(NMePSde) -> Mux/30
  Rule Set/38(NSePMde) -> Mux/38
  Rule Set/22(NBeZde) -> Mux/22
  Rule Set/21(PBeNSde) -> Mux/21
  Rule Set/20(PMeNSde) -> Mux/20
  Rule Set/15(NBeNSde) -> Mux/15
  Rule Set/12(PSeNMde) -> Mux/12
  Rule Set/8(NBeNMde) -> Mux/8
  Rule Set/7(PBeNBde) -> Mux/7
  Rule Set/3(NSeNBde) -> Mux/3
  Rule Set/1(NBeNBde) -> Mux/1
  Rule Set/19(PSeNSde) -> Mux/19
  Rule Set/4(ZeNBde) -> Mux/4
  Rule Set/18(ZeNSde) -> Mux/18
  Rule Set/17(NSeNSde) -> Mux/17
  Rule Set/13(PMeNMde) -> Mux/13
  Rule Set/11(ZeNMde) -> Mux/11
  Rule Set/16(NMeNSde) -> Mux/16
  Rule Set/14(PBeNMde) -> Mux/14
  Rule Set/6(PMeNBde) -> Mux/6
  Rule Set/10(NSeNMde) -> Mux/10
  Rule Set/9(NMeNMde) -> Mux/9
  Rule Set/5(PSeNBde) -> Mux/5
  Rule Set/2(NMeNBde) -> Mux/2
  PMe/1 -> Rule Set/6(PMe)
  NSe/1 -> Rule Set/3(NSe)
  Ze/1 -> Rule Set/4(Ze)
  NSde/1 -> Rule Set/10(NSde)
  PBde/1 -> Rule Set/14(PBde)
  NMe/1 -> Rule Set/2(NMe)
  NBde/1 -> Rule Set/8(NBde)
  PSe/1 -> Rule Set/5(PSe)
  PMde/1 -> Rule Set/13(PMde)
  PSde/1 -> Rule Set/12(PSde)
  Zde/1 -> Rule Set/11(Zde)
  NMde/1 -> Rule Set/9(NMde)
  PBe/1 -> Rule Set/7(PBe)
  NBe/1 -> Rule Set/1(NBe)
  Ki Defuzzyfication/1(Out1) -> Ki fuzzy/1
  k1 Defuzzyfication/1(Out1) -> k1/1
  k2 Defuzzyfication/1(Out1) -> k2/1
  k3 Defuzzyfication/1(Out1) -> k3/1

== system PII_speed/FGS SSC/FGS/TF calc ==
  Kif : Inport
  k1f : Inport  Port=2
  k2f : Inport  Port=3
  k3f : Inport  Port=4
  MATLAB Function : Stateflow chart  TreatAsAtomicUnit=on
  L : Outport
  M : Outport  Port=2
  wires:
  MATLAB Function/2(M) -> M/1
  MATLAB Function/1(L) -> L/1
  [T2] -> MATLAB Function/5(T2)
  [Tc] -> MATLAB Function/6(Tc)
  k2f/1 -> MATLAB Function/3(k2f)
  k1f/1 -> MATLAB Function/2(k1f)
  Kif/1 -> MATLAB Function/1(Kif)
  k3f/1 -> MATLAB Function/4(k3f)

== system PII_speed/RTI Data/RTI Data Store/RTI Data Store ==
  RTI Data Store : Subsystem
      mask Type: RTI_DATA_STORE
      mask Description:
      | RTI Data Store Block. This block is used by RTI to store internal model dependent data. Deleting this block will result in data loss.
      | 
      | NEVER DELETE, COPY, OR MODIFY THIS BLOCK!
      mask Help:
      | RTI Data Store Block. This block is used by RTI to store internal model dependent data. Deleting this block will result in data loss.
      | 
      | NEVER DELETE, COPY, OR MODIFY THIS BLOCK!
      mask Display: text(0.5, 0.5, ' ', 'HorizontalAlignment', 'center');

== system PII_speed/FGS SSC/FGS/Rule Set & Defuzzyfication/Ki Defuzzyfication ==
  In1 : Inport
  Demux : Demux  Outputs=49
  Subsystem3 : Subsystem
  Out1 : Outport
  wires:
  Demux/30 -> Subsystem3/30(In30)
  Demux/28 -> Subsystem3/28(In28)
  Demux/29 -> Subsystem3/29(In29)
  Demux/18 -> Subsystem3/18(In18)
  Demux/31 -> Subsystem3/31(In31)
  Demux/22 -> Subsystem3/22(In22)
  Demux/23 -> Subsystem3/23(In23)
  Demux/20 -> Subsystem3/20(In20)
  Demux/19 -> Subsystem3/19(In19)
  Demux/10 -> Subsystem3/10(In10)
  Demux/15 -> Subsystem3/15(In15)
  Demux/25 -> Subsystem3/25(In25)
  Demux/32 -> Subsystem3/32(In32)
  Demux/24 -> Subsystem3/24(In24)
  Demux/21 -> Subsystem3/21(In21)
  Demux/4 -> Subsystem3/4(In4)
  Demux/13 -> Subsystem3/13(In13)
  Demux/5 -> Subsystem3/5(In5)
  Demux/6 -> Subsystem3/6(In6)
  Demux/17 -> Subsystem3/17(In17)
  Demux/16 -> Subsystem3/16(In16)
  Demux/14 -> Subsystem3/14(In14)
  Demux/11 -> Subsystem3/11(In11)
  Demux/12 -> Subsystem3/12(In12)
  Demux/9 -> Subsystem3/9(In9)
  Demux/8 -> Subsystem3/8(In8)
  Demux/3 -> Subsystem3/3(In3)
  Demux/7 -> Subsystem3/7(In7)
  In1/1 -> Demux/1
  Subsystem3/1(Out1) -> Out1/1
  Demux/40 -> Subsystem3/40(In40)
  Demux/43 -> Subsystem3/43(In43)
  Demux/49 -> Subsystem3/49(In49)
  Demux/46 -> Subsystem3/46(In46)
  Demux/42 -> Subsystem3/42(In42)
  Demux/39 -> Subsystem3/39(In39)
  Demux/36 -> Subsystem3/36(In36)
  Demux/48 -> Subsystem3/48(In48)
  Demux/26 -> Subsystem3/26(In26)
  Demux/37 -> Subsystem3/37(In37)
  Demux/44 -> Subsystem3/44(In44)
  Demux/45 -> Subsystem3/45(In45)
  Demux/41 -> Subsystem3/41(In41)
  Demux/27 -> Subsystem3/27(In27)
  Demux/34 -> Subsystem3/34(In34)
  Demux/33 -> Subsystem3/33(In33)
  Demux/47 -> Subsystem3/47(In47)
  Demux/2 -> Subsystem3/2(In2)
  Demux/38 -> Subsystem3/38(In38)
  Demux/35 -> Subsystem3/35(In35)
  Demux/1 -> Subsystem3/1(In1)

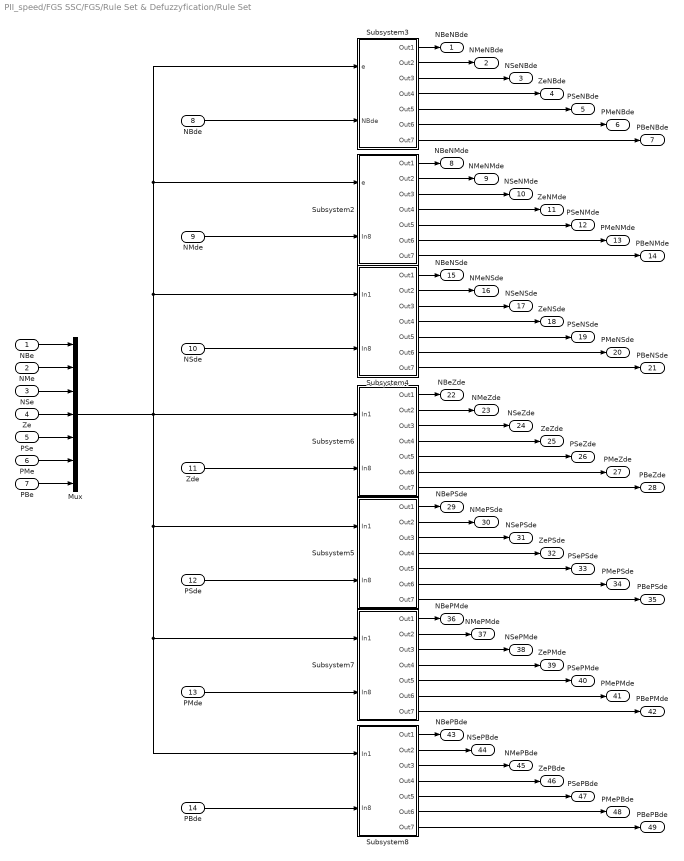
== system PII_speed/FGS SSC/FGS/Rule Set & Defuzzyfication/Rule Set ==
  NBe : Inport
  NMe : Inport  Port=2
  NSe : Inport  Port=3
  Ze : Inport  Port=4
  PSe : Inport  Port=5
  PMe : Inport  Port=6
  PBe : Inport  Port=7
  NBde : Inport  Port=8
  NMde : Inport  Port=9
  NSde : Inport  Port=10
  Zde : Inport  Port=11
  PSde : Inport  Port=12
  PMde : Inport  Port=13
  PBde : Inport  Port=14
  Mux : Mux  Inputs=7
  Subsystem2 : Subsystem
  Subsystem3 : Subsystem
  Subsystem4 : Subsystem
  Subsystem5 : Subsystem
  Subsystem6 : Subsystem
  Subsystem7 : Subsystem
  Subsystem8 : Subsystem
  NBeNBde : Outport
  NMeNBde : Outport  Port=2
  NSeNBde : Outport  Port=3
  ZeNBde : Outport  Port=4
  PSeNBde : Outport  Port=5
  PMeNBde : Outport  Port=6
  PBeNBde : Outport  Port=7
  NBeNMde : Outport  Port=8
  NMeNMde : Outport  Port=9
  NSeNMde : Outport  Port=10
  ZeNMde : Outport  Port=11
  PSeNMde : Outport  Port=12
  PMeNMde : Outport  Port=13
  PBeNMde : Outport  Port=14
  NBeNSde : Outport  Port=15
  NMeNSde : Outport  Port=16
  NSeNSde : Outport  Port=17
  ZeNSde : Outport  Port=18
  PSeNSde : Outport  Port=19
  PMeNSde : Outport  Port=20
  PBeNSde : Outport  Port=21
  NBeZde : Outport  Port=22
  NMeZde : Outport  Port=23
  NSeZde : Outport  Port=24
  ZeZde : Outport  Port=25
  PSeZde : Outport  Port=26
  PMeZde : Outport  Port=27
  PBeZde : Outport  Port=28
  NBePSde : Outport  Port=29
  NMePSde : Outport  Port=30
  NSePSde : Outport  Port=31
  ZePSde : Outport  Port=32
  PSePSde : Outport  Port=33
  PMePSde : Outport  Port=34
  PBePSde : Outport  Port=35
  NBePMde : Outport  Port=36
  NMePMde : Outport  Port=37
  NSePMde : Outport  Port=38
  ZePMde : Outport  Port=39
  PSePMde : Outport  Port=40
  PMePMde : Outport  Port=41
  PBePMde : Outport  Port=42
  NBePBde : Outport  Port=43
  NSePBde : Outport  Port=44
  NMePBde : Outport  Port=45
  ZePBde : Outport  Port=46
  PSePBde : Outport  Port=47
  PMePBde : Outport  Port=48
  PBePBde : Outport  Port=49
  wires:
  Subsystem8/4(Out4) -> ZePBde/1
  Subsystem8/1(Out1) -> NBePBde/1
  Subsystem7/7(Out7) -> PBePMde/1
  Subsystem7/6(Out6) -> PMePMde/1
  Subsystem7/2(Out2) -> NMePMde/1
  Subsystem5/4(Out4) -> ZePSde/1
  Subsystem6/1(Out1) -> NBeZde/1
  Subsystem5/6(Out6) -> PMePSde/1
  Subsystem6/4(Out4) -> ZeZde/1
  Subsystem5/5(Out5) -> PSePSde/1
  Subsystem6/3(Out3) -> NSeZde/1
  Subsystem7/3(Out3) -> NSePMde/1
  Subsystem5/2(Out2) -> NMePSde/1
  Subsystem8/7(Out7) -> PBePBde/1
  Subsystem5/1(Out1) -> NBePSde/1
  Subsystem8/6(Out6) -> PMePBde/1
  Subsystem8/5(Out5) -> PSePBde/1
  Subsystem4/7(Out7) -> PBeNSde/1
  Subsystem7/5(Out5) -> PSePMde/1
  Subsystem8/3(Out3) -> NMePBde/1
  Subsystem5/7(Out7) -> PBePSde/1
  Subsystem8/2(Out2) -> NSePBde/1
  Subsystem5/3(Out3) -> NSePSde/1
  Subsystem6/6(Out6) -> PMeZde/1
  Subsystem7/1(Out1) -> NBePMde/1
  Subsystem7/4(Out4) -> ZePMde/1
  Subsystem6/7(Out7) -> PBeZde/1
  Subsystem6/2(Out2) -> NMeZde/1
  Subsystem6/5(Out5) -> PSeZde/1
  Subsystem2/4(Out4) -> ZeNMde/1
  Subsystem2/5(Out5) -> PSeNMde/1
  Subsystem3/6(Out6) -> PMeNBde/1
  PMe/1 -> Mux/6
  Subsystem4/6(Out6) -> PMeNSde/1
  Subsystem4/2(Out2) -> NMeNSde/1
  Subsystem4/1(Out1) -> NBeNSde/1
  Subsystem2/1(Out1) -> NBeNMde/1
  NBe/1 -> Mux/1
  PMde/1 -> Subsystem7/2(In8)
  Subsystem2/2(Out2) -> NMeNMde/1
  PSe/1 -> Mux/5
  PBe/1 -> Mux/7
  Subsystem2/3(Out3) -> NSeNMde/1
  Subsystem3/5(Out5) -> PSeNBde/1
  Subsystem3/2(Out2) -> NMeNBde/1
  Subsystem4/5(Out5) -> PSeNSde/1
  PSde/1 -> Subsystem5/2(In8)
  Zde/1 -> Subsystem6/2(In8)
  NMe/1 -> Mux/2
  Subsystem3/7(Out7) -> PBeNBde/1
  PBde/1 -> Subsystem8/2(In8)
  Ze/1 -> Mux/4
  NSe/1 -> Mux/3
  Subsystem4/4(Out4) -> ZeNSde/1
  Subsystem3/3(Out3) -> NSeNBde/1
  Subsystem4/3(Out3) -> NSeNSde/1
  Subsystem2/7(Out7) -> PBeNMde/1
  Mux/1 -> Subsystem6/1(In1), Subsystem8/1(In1), Subsystem7/1(In1), Subsystem5/1(In1), Subsystem4/1(In1), Subsystem3/1(e), Subsystem2/1(e)
  Subsystem3/1(Out1) -> NBeNBde/1
  Subsystem2/6(Out6) -> PMeNMde/1
  Subsystem3/4(Out4) -> ZeNBde/1
  NSde/1 -> Subsystem4/2(In8)
  NBde/1 -> Subsystem3/2(NBde)
  NMde/1 -> Subsystem2/2(In8)

== system PII_speed/FGS SSC/FGS/Rule Set & Defuzzyfication/k1 Defuzzyfication ==
  In1 : Inport
  Demux : Demux  Outputs=49
  Subsystem3 : Subsystem
  Out1 : Outport
  wires:
  Demux/1 -> Subsystem3/1(In1)
  Demux/35 -> Subsystem3/35(In35)
  Demux/38 -> Subsystem3/38(In38)
  Demux/2 -> Subsystem3/2(In2)
  Demux/47 -> Subsystem3/47(In47)
  Demux/33 -> Subsystem3/33(In33)
  Demux/34 -> Subsystem3/34(In34)
  Demux/27 -> Subsystem3/27(In27)
  Demux/41 -> Subsystem3/41(In41)
  Demux/45 -> Subsystem3/45(In45)
  Demux/44 -> Subsystem3/44(In44)
  Demux/37 -> Subsystem3/37(In37)
  Demux/26 -> Subsystem3/26(In26)
  Demux/48 -> Subsystem3/48(In48)
  Demux/36 -> Subsystem3/36(In36)
  Demux/39 -> Subsystem3/39(In39)
  Demux/42 -> Subsystem3/42(In42)
  Demux/46 -> Subsystem3/46(In46)
  Demux/49 -> Subsystem3/49(In49)
  Demux/43 -> Subsystem3/43(In43)
  Demux/40 -> Subsystem3/40(In40)
  Subsystem3/1(Out1) -> Out1/1
  In1/1 -> Demux/1
  Demux/7 -> Subsystem3/7(In7)
  Demux/3 -> Subsystem3/3(In3)
  Demux/8 -> Subsystem3/8(In8)
  Demux/9 -> Subsystem3/9(In9)
  Demux/12 -> Subsystem3/12(In12)
  Demux/11 -> Subsystem3/11(In11)
  Demux/14 -> Subsystem3/14(In14)
  Demux/16 -> Subsystem3/16(In16)
  Demux/17 -> Subsystem3/17(In17)
  Demux/6 -> Subsystem3/6(In6)
  Demux/5 -> Subsystem3/5(In5)
  Demux/13 -> Subsystem3/13(In13)
  Demux/4 -> Subsystem3/4(In4)
  Demux/21 -> Subsystem3/21(In21)
  Demux/24 -> Subsystem3/24(In24)
  Demux/32 -> Subsystem3/32(In32)
  Demux/25 -> Subsystem3/25(In25)
  Demux/15 -> Subsystem3/15(In15)
  Demux/10 -> Subsystem3/10(In10)
  Demux/19 -> Subsystem3/19(In19)
  Demux/20 -> Subsystem3/20(In20)
  Demux/23 -> Subsystem3/23(In23)
  Demux/22 -> Subsystem3/22(In22)
  Demux/31 -> Subsystem3/31(In31)
  Demux/18 -> Subsystem3/18(In18)
  Demux/29 -> Subsystem3/29(In29)
  Demux/28 -> Subsystem3/28(In28)
  Demux/30 -> Subsystem3/30(In30)

== system PII_speed/FGS SSC/FGS/Rule Set & Defuzzyfication/k2 Defuzzyfication ==
  In1 : Inport
  Demux2 : Demux  Outputs=49
  Subsystem2 : Subsystem
  Out1 : Outport
  wires:
  Demux2/26 -> Subsystem2/26(In26)
  Demux2/25 -> Subsystem2/25(In25)
  Subsystem2/1(Out1) -> Out1/1
  In1/1 -> Demux2/1
  Demux2/20 -> Subsystem2/20(In20)
  Demux2/32 -> Subsystem2/32(In32)
  Demux2/8 -> Subsystem2/8(In8)
  Demux2/19 -> Subsystem2/19(In19)
  Demux2/30 -> Subsystem2/30(In30)
  Demux2/31 -> Subsystem2/31(In31)
  Demux2/27 -> Subsystem2/27(In27)
  Demux2/23 -> Subsystem2/23(In23)
  Demux2/1 -> Subsystem2/1(In1)
  Demux2/3 -> Subsystem2/3(In3)
  Demux2/5 -> Subsystem2/5(In5)
  Demux2/7 -> Subsystem2/7(In7)
  Demux2/28 -> Subsystem2/28(In28)
  Demux2/17 -> Subsystem2/17(In17)
  Demux2/18 -> Subsystem2/18(In18)
  Demux2/9 -> Subsystem2/9(In9)
  Demux2/29 -> Subsystem2/29(In29)
  Demux2/4 -> Subsystem2/4(In4)
  Demux2/6 -> Subsystem2/6(In6)
  Demux2/2 -> Subsystem2/2(In2)
  Demux2/22 -> Subsystem2/22(In22)
  Demux2/24 -> Subsystem2/24(In24)
  Demux2/21 -> Subsystem2/21(In21)
  Demux2/36 -> Subsystem2/36(In36)
  Demux2/14 -> Subsystem2/14(In14)
  Demux2/33 -> Subsystem2/33(In33)
  Demux2/47 -> Subsystem2/47(In47)
  Demux2/37 -> Subsystem2/37(In37)
  Demux2/12 -> Subsystem2/12(In12)
  Demux2/13 -> Subsystem2/13(In13)
  Demux2/11 -> Subsystem2/11(In11)
  Demux2/44 -> Subsystem2/44(In44)
  Demux2/41 -> Subsystem2/41(In41)
  Demux2/43 -> Subsystem2/43(In43)
  Demux2/45 -> Subsystem2/45(In45)
  Demux2/10 -> Subsystem2/10(In10)
  Demux2/38 -> Subsystem2/38(In38)
  Demux2/42 -> Subsystem2/42(In42)
  Demux2/49 -> Subsystem2/49(In49)
  Demux2/48 -> Subsystem2/48(In48)
  Demux2/34 -> Subsystem2/34(In34)
  Demux2/46 -> Subsystem2/46(In46)
  Demux2/35 -> Subsystem2/35(In35)
  Demux2/39 -> Subsystem2/39(In39)
  Demux2/40 -> Subsystem2/40(In40)
  Demux2/15 -> Subsystem2/15(In15)
  Demux2/16 -> Subsystem2/16(In16)

== system PII_speed/FGS SSC/FGS/Rule Set & Defuzzyfication/k3 Defuzzyfication ==
  In1 : Inport
  Demux2 : Demux  Outputs=49
  Subsystem2 : Subsystem
  Out1 : Outport
  wires:
  Demux2/16 -> Subsystem2/16(In16)
  Demux2/15 -> Subsystem2/15(In15)
  Demux2/40 -> Subsystem2/40(In40)
  Demux2/39 -> Subsystem2/39(In39)
  Demux2/35 -> Subsystem2/35(In35)
  Demux2/46 -> Subsystem2/46(In46)
  Demux2/34 -> Subsystem2/34(In34)
  Demux2/48 -> Subsystem2/48(In48)
  Demux2/49 -> Subsystem2/49(In49)
  Demux2/42 -> Subsystem2/42(In42)
  Demux2/38 -> Subsystem2/38(In38)
  Demux2/10 -> Subsystem2/10(In10)
  Demux2/45 -> Subsystem2/45(In45)
  Demux2/43 -> Subsystem2/43(In43)
  Demux2/41 -> Subsystem2/41(In41)
  Demux2/44 -> Subsystem2/44(In44)
  Demux2/11 -> Subsystem2/11(In11)
  Demux2/13 -> Subsystem2/13(In13)
  Demux2/12 -> Subsystem2/12(In12)
  Demux2/37 -> Subsystem2/37(In37)
  Demux2/47 -> Subsystem2/47(In47)
  Demux2/33 -> Subsystem2/33(In33)
  Demux2/14 -> Subsystem2/14(In14)
  Demux2/36 -> Subsystem2/36(In36)
  Demux2/21 -> Subsystem2/21(In21)
  Demux2/24 -> Subsystem2/24(In24)
  Demux2/22 -> Subsystem2/22(In22)
  Demux2/2 -> Subsystem2/2(In2)
  Demux2/6 -> Subsystem2/6(In6)
  Demux2/4 -> Subsystem2/4(In4)
  Demux2/29 -> Subsystem2/29(In29)
  Demux2/9 -> Subsystem2/9(In9)
  Demux2/18 -> Subsystem2/18(In18)
  Demux2/17 -> Subsystem2/17(In17)
  Demux2/28 -> Subsystem2/28(In28)
  Demux2/7 -> Subsystem2/7(In7)
  Demux2/5 -> Subsystem2/5(In5)
  Demux2/3 -> Subsystem2/3(In3)
  Demux2/1 -> Subsystem2/1(In1)
  Demux2/23 -> Subsystem2/23(In23)
  Demux2/27 -> Subsystem2/27(In27)
  Demux2/31 -> Subsystem2/31(In31)
  Demux2/30 -> Subsystem2/30(In30)
  Demux2/19 -> Subsystem2/19(In19)
  Demux2/8 -> Subsystem2/8(In8)
  Demux2/32 -> Subsystem2/32(In32)
  Demux2/20 -> Subsystem2/20(In20)
  In1/1 -> Demux2/1
  Subsystem2/1(Out1) -> Out1/1
  Demux2/25 -> Subsystem2/25(In25)
  Demux2/26 -> Subsystem2/26(In26)

== system PII_speed/RTI Data/RTI Data Store/RTI Data Store/RTI Data Store ==
  RTI Data Store : Subsystem
      mask Type: RTI_DATA_STORE
      mask Description:
      | RTI Data Store Block. This block is used by RTI to store internal model dependent data. Deleting this block will result in data loss.
      | 
      | NEVER DELETE, COPY, OR MODIFY THIS BLOCK!
      mask Help:
      | RTI Data Store Block. This block is used by RTI to store internal model dependent data. Deleting this block will result in data loss.
      | 
      | NEVER DELETE, COPY, OR MODIFY THIS BLOCK!
      mask Display: text(0.5, 0.5, ' ', 'HorizontalAlignment', 'center');
